simulink model "visualizacionsonar"  (R2023b)
settings: Solver=VariableStepAuto  StartTime=0.0  StopTime=10.0  RelTol=1e-3
libraries: arduinolib x2
settings Model: Creator=Usuario_UMA  LastModifiedBy=Usuario_UMA

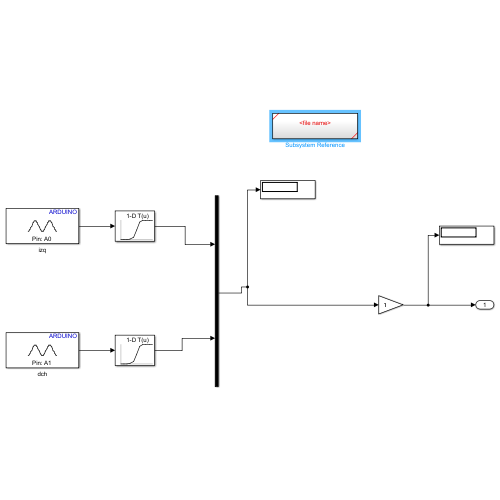
[thumbnail: Simulink's stored preview of the top-level diagram]
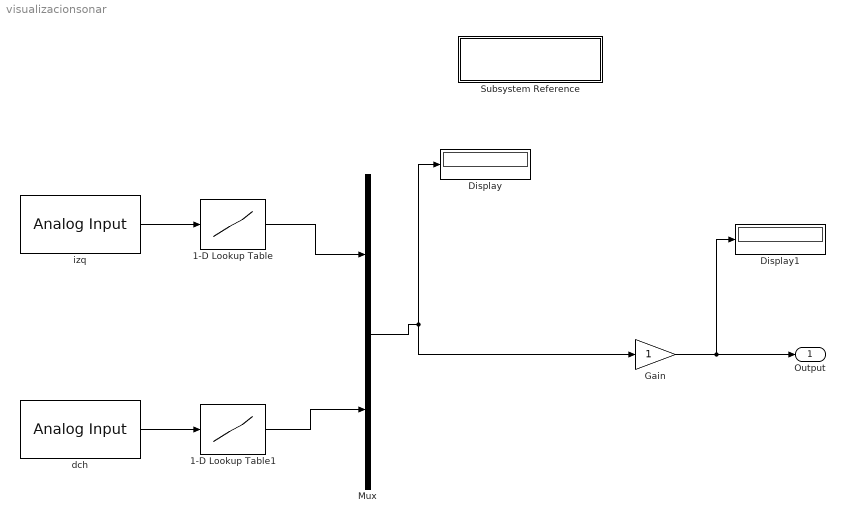
== system visualizacionsonar ==
  1-D Lookup Table : Lookup_n-D  NumberOfTableDimensions=1  BreakpointsForDimension1=[-5:5]  Table=tanh([-5:5])  InternalRulePriority=Speed  RndMeth=Simplest
  1-D Lookup Table1 : Lookup_n-D  NumberOfTableDimensions=1  BreakpointsForDimension1=[-5:5]  Table=tanh([-5:5])  InternalRulePriority=Speed  RndMeth=Simplest
  Display : Display
  Display1 : Display
  Gain : Gain
  Mux : Mux  Inputs=2
  Subsystem Reference : Subsystem  ReferencedSubsystem=<file name>
  dch : arduinolib/Analog Input  pinNumber=1  ReadResultsOnly=off  ConversionTriggerSource=Software  ExternalTriggerType=uint32( 0 )  OutputDataType=uint16  EnableConversionCompleteNotify=off  EnableOuputStatus=off  SampleTime=-1  blockPlatform=arduino
  izq : arduinolib/Analog Input  pinNumber=0  ReadResultsOnly=off  ConversionTriggerSource=Software  ExternalTriggerType=uint32( 0 )  OutputDataType=uint16  EnableConversionCompleteNotify=off  EnableOuputStatus=off  SampleTime=-1  blockPlatform=arduino
  Output : Outport
  wires:
  Mux/1 -> Gain/1, Display/1
  Gain/1 -> Display1/1, Output/1
  dch/1 -> 1-D Lookup Table1/1
  1-D Lookup Table1/1 -> Mux/2
  izq/1 -> 1-D Lookup Table/1
  1-D Lookup Table/1 -> Mux/1

== system visualizacionsonar/Subsystem Reference ==
